simulink subsystem "find_ti_index"  (R2021b)
settings: Solver=VariableStepAuto  StartTime=0.0  StopTime=10.0  RelTol=1e-3
undefined symbols (not defined in the file): req_mem_size
settings Model: Creator=torha  LastModifiedBy=torha
settings SolverCC: AlgebraicLoopSolver=TrustRegion
settings DebuggingCC: SFMachineParentedDataDiag=warning

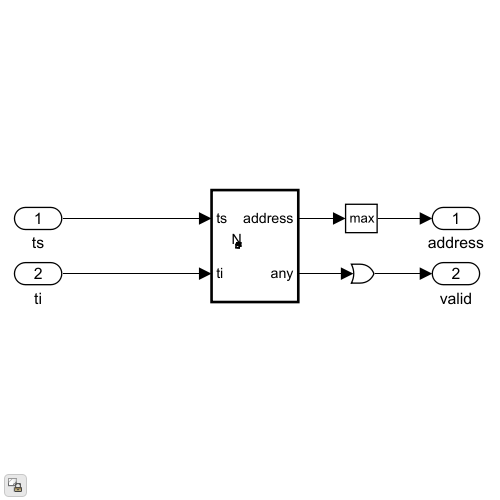
[thumbnail: Simulink's stored preview of the top-level diagram]
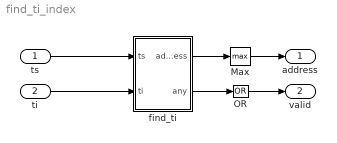
== system find_ti_index ==
  ts : Inport
  ti : Inport  Port=2
  Max : MinMax  Function=max
  OR : Logic  Operator=OR  Inputs=1  IconShape=distinctive  AllPortsSameDT=off  OutDataTypeStr=boolean
  find_ti : Subsystem  mask{iter=fi(0:req_mem_size-1, false, log2(req_mem_size), 0)}
  address : Outport
  valid : Outport  Port=2
  wires:
  OR/1 -> valid/1
  Max/1 -> address/1
  ts/1 -> find_ti/1(ts)
  find_ti/2(any) -> OR/1
  ti/1 -> find_ti/2(ti)
  find_ti/1(address) -> Max/1

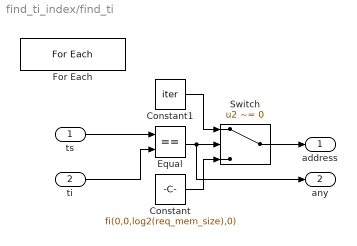
== system find_ti_index/find_ti ==
  ts : Inport  Partition=on  PartitionDimension=1  PartitionWidth=1  PartitionOffset=0
  ti : Inport  Port=2
  Constant : Constant  Value=fi(0,0,log2(req_mem_size),0)
  Constant1 : Constant  Value=iter
  Equal : RelationalOperator  Operator===  OutDataTypeStr=boolean  RndMeth=Simplest
  For Each : ForEach  DisableCoverage=on  IterateSubsysMaskParameter=on  SubsysMaskParameterIterationDimension=2
  Switch : Switch  Criteria=u2 ~= 0
  address : Outport  ConcatenationDimension=1
  any : Outport  Port=2  ConcatenationDimension=1
  wires:
  ti/1 -> Equal/2
  ts/1 -> Equal/1
  Switch/1 -> address/1
  Equal/1 -> Switch/2, any/1
  Constant/1 -> Switch/3
  Constant1/1 -> Switch/1
